simulink model "CLIK_II_ordine"  (R2023a)
settings: Solver=VariableStepAuto  StartTime=0.0  StopTime=113  RelTol=1e-3
values from neighbouring files (symbols this model uses):
  a1 = 0.5    [Progetto_FoR.m]
  d0 = 1    [Progetto_FoR.m]
  KD = diag(kd)    [Progetto_FoR.m]
  KP = diag(kp)    [Progetto_FoR.m]
  q0 = [0 pi/2 0 pi/2]    [Progetto_FoR.m]
  Tc = 0.001    [Progetto_FoR.m]
undefined symbols (not defined in the file or in its folder): DiscIntNeverNeededParam
settings Model: Creator=panto  LastModifiedBy=panto

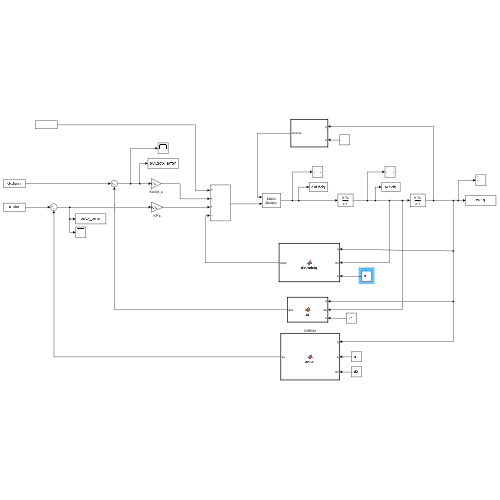
[thumbnail: Simulink's stored preview of the top-level diagram]
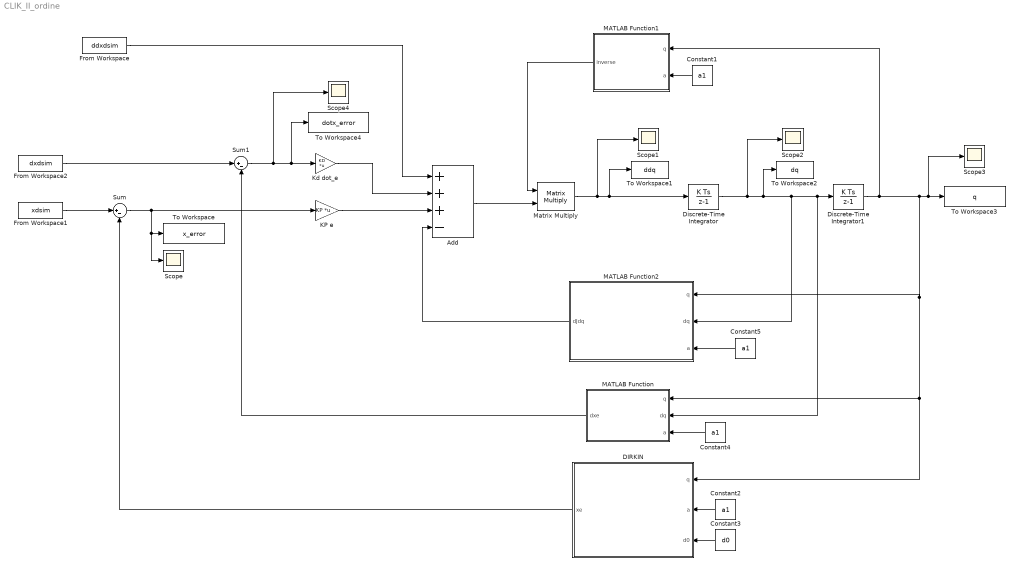
== system CLIK_II_ordine ==
  Add : Sum  Inputs=+++-
  Constant{1..2,4..5} (4 alike) : Constant  Value=a1
  Constant3 : Constant  Value=d0
  DIRKIN : MATLAB Function  TreatAsAtomicUnit=on
  Discrete-Time Integrator : DiscreteIntegrator  SampleTime=Tc  ICPrevOutput=DiscIntNeverNeededParam  ICPrevScaledInput=DiscIntNeverNeededParam
  Discrete-Time Integrator1 : DiscreteIntegrator  InitialCondition=q0'  SampleTime=Tc  ICPrevOutput=DiscIntNeverNeededParam  ICPrevScaledInput=DiscIntNeverNeededParam
  From Workspace : FromWorkspace  VariableName=ddxdsim  SampleTime=Tc
  From Workspace1 : FromWorkspace  VariableName=xdsim  SampleTime=Tc
  From Workspace2 : FromWorkspace  VariableName=dxdsim  SampleTime=Tc
  KP e : Gain  Gain=KP  Multiplication=Matrix(K*u)
  Kd dot_e : Gain  Gain=KD  Multiplication=Matrix(K*u)
  MATLAB Function : MATLAB Function  TreatAsAtomicUnit=on
  MATLAB Function1 : MATLAB Function  TreatAsAtomicUnit=on
  MATLAB Function2 : MATLAB Function  TreatAsAtomicUnit=on
  Matrix Multiply : Product  Multiplication=Matrix(*)
  Scope{,1..4} (5 alike) : Scope
  Sum : Sum  Inputs=|+-
  Sum1 : Sum  Inputs=|+-
  To Workspace : ToWorkspace  VariableName=x_error  SampleTime=Tc
      settings: Save2DSignal=2-D array (concatenate along first dimension)
  To Workspace1 : ToWorkspace  VariableName=ddq  SampleTime=-1
      settings: Save2DSignal=2-D array (concatenate along first dimension)
  To Workspace2 : ToWorkspace  VariableName=dq  SampleTime=-1
      settings: Save2DSignal=2-D array (concatenate along first dimension)
  To Workspace3 : ToWorkspace  VariableName=q  SampleTime=Tc
      settings: Save2DSignal=2-D array (concatenate along first dimension)
  To Workspace4 : ToWorkspace  VariableName=dotx_error  SampleTime=-1
      settings: Save2DSignal=2-D array (concatenate along first dimension)
  wires:
  Constant2/1 -> DIRKIN/2(a)
  Constant3/1 -> DIRKIN/3(d0)
  From Workspace1/1 -> Sum/1
  Sum/1 -> Scope/1, To Workspace/1, KP e/1
  DIRKIN/1(xe) -> Sum/2
  Kd dot_e/1 -> Add/2
  Add/1 -> Matrix Multiply/2
  Matrix Multiply/1 -> Scope1/1, To Workspace1/1, Discrete-Time Integrator/1
  Discrete-Time Integrator/1 -> Scope2/1, To Workspace2/1, MATLAB Function2/2(dq), MATLAB Function/2(dq), Discrete-Time Integrator1/1
  Discrete-Time Integrator1/1 -> MATLAB Function2/1(q), MATLAB Function/1(q), DIRKIN/1(q), Scope3/1, To Workspace3/1, MATLAB Function1/1(q)
  Constant1/1 -> MATLAB Function1/2(a)
  MATLAB Function1/1(inverse) -> Matrix Multiply/1
  From Workspace2/1 -> Sum1/1
  KP e/1 -> Add/3
  Sum1/1 -> Scope4/1, To Workspace4/1, Kd dot_e/1
  From Workspace/1 -> Add/1
  Constant4/1 -> MATLAB Function/3(a)
  MATLAB Function/1(dxe) -> Sum1/2
  MATLAB Function2/1(dJdq) -> Add/4
  Constant5/1 -> MATLAB Function2/3(a)

== matlab function CLIK_II_ordine/MATLAB Function1 ==
  data: q input; inverse output; a input
function inverse = invJ(q,a)
%devo prima calcolare lo Jacobiano analitico e poi invertirlo
%Nel caso dello SCARA, lo Jacobiano analitico coincide con quello
%geometrico: questo perchè nello SCARA l'orientamento può essere
%rappresentato direttamente dall'angolo attorno a z, e quindi la velocità
%angolare z si traduce direttamente nella velocità di cambiamento
%dell'angolo di orientamento attorno z
%dal libro when the DOFs cause rotations of the end-effector all about the 
% same fixed axis in space, the two Jacobians are essentially the same
   
    Ja = zeros(4,4);
    Ja = [-a*sin(q(1)+q(2))-a*sin(q(1)) -a*sin(q(1)+q(2)) 0 0;
        a*cos(q(1)+q(2))+a*cos(q(1)) a*cos(q(1)+q(2)) 0 0;
        0 0 -1 0;
        1 1 0 -1];

    inverse = inv(Ja);

end

== matlab function CLIK_II_ordine/DIRKIN ==
  data: q input; xe output; a input; d0 input
function xe = dirkyn(q, a, d0)
  xe = zeros(4,1);
    xe = [a*cos(q(1)+q(2))+a*cos(q(1));
        a*sin(q(1)+q(2))+a*sin(q(1));
        d0-q(3);
        q(1)+q(2)-q(4)];
end

== matlab function CLIK_II_ordine/MATLAB Function ==
  data: q input; dq input; dxe output; a input
function dxe = Ja(q,dq,a)

Ja = zeros(4,4);
Ja = [-a*sin(q(1)+q(2))-a*sin(q(1)) -a*sin(q(1)+q(2)) 0 0;
        a*cos(q(1)+q(2))+a*cos(q(1)) a*cos(q(1)+q(2)) 0 0;
        0 0 -1 0;
        1 1 0 -1];

    dxe = Ja*dq;

end

== matlab function CLIK_II_ordine/MATLAB Function2 ==
  data: q input; dq input; dJdq output; a input
function dJdq =  dotJadotq(q,dq,a)
    
    dotJa = zeros(4,4);
    dotJa = [-a*cos(q(1))*dq(1)-a*cos(q(1)+q(2))*(dq(1)+dq(2)) -a*cos(q(1)+q(2))*(dq(1)+dq(2)) 0 0;
        -a*sin(q(1))*dq(1)-a*sin(q(1)+q(2))*(dq(1)+dq(2)) -a*sin(q(1)+q(2))*(dq(1)+dq(2)) 0 0;
        0 0 0 0;
        0 0 0 0];

    dJdq = dotJa*dq;

end
